simulink model "CrawlerValidation_Backup"  (R2018b)
settings: Solver=VariableStepAuto  StartTime=0.0  StopTime=10.0  RelTol=1e-3
model workspace: external: MAT-File C:\CrawlerValidation_DataFile1.mat (data not in the file)
undefined symbols (not defined in the file): smiData, X, Y, Z
libraries: sm_lib x20, nesl_utility x7
settings Model: Creator=Kim Jensen  LastModifiedBy=Kim Jensen

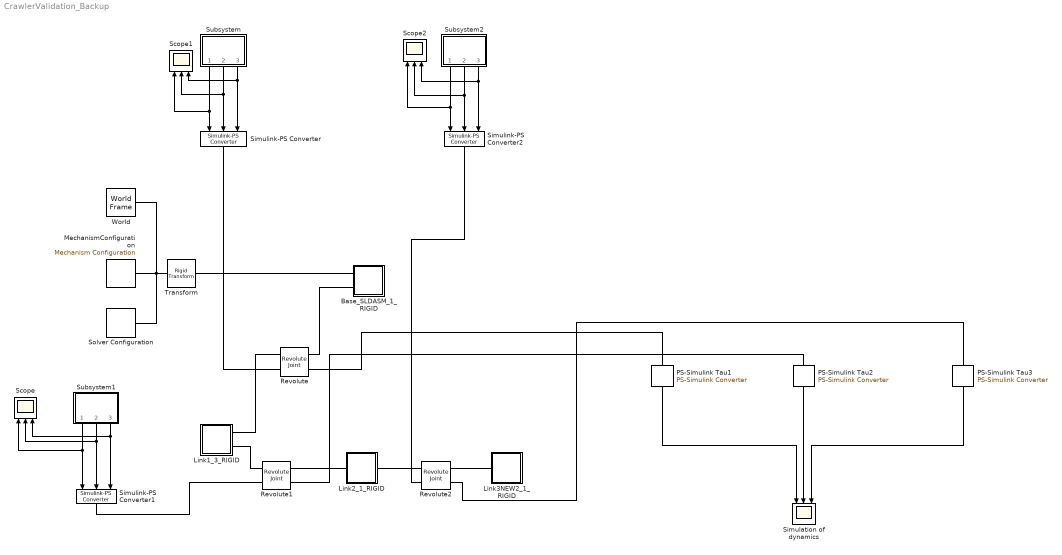
== system CrawlerValidation_Backup ==
  Base_SLDASM_1_RIGID : Subsystem
  Link1_3_RIGID : Subsystem
  Link2_1_RIGID : Subsystem
  Link3NEW2_1_RIGID : Subsystem
  MechanismConfiguration : sm_lib/Utilities/Mechanism Configuration  UniformGravity=Constant  GravityVector=[0 -9.80665 0]  GravityUnits=m/s^2  LinearizationDelta=0.001
  PS-Simulink Tau1 : nesl_utility/PS-Simulink Converter  PhysicalDomain=network_engine_domain  SubClassName=ps_output  LeftPortType=input  RightPortType=output  PseudoPeriodic=off  Frequencies=[]  Unit=1  AffineConversion=off
  PS-Simulink Tau2 : nesl_utility/PS-Simulink Converter  PhysicalDomain=network_engine_domain  SubClassName=ps_output  LeftPortType=input  RightPortType=output  PseudoPeriodic=off  Frequencies=[]  Unit=1  AffineConversion=off
  PS-Simulink Tau3 : nesl_utility/PS-Simulink Converter  PhysicalDomain=network_engine_domain  SubClassName=ps_output  LeftPortType=input  RightPortType=output  PseudoPeriodic=off  Frequencies=[]  Unit=1  AffineConversion=off
  Revolute : sm_lib/Joints/Revolute Joint  SenseConstraintForce=off  SenseConstraintForceX=off  SenseConstraintForceY=off  SenseConstraintForceZ=off  SenseConstraintTorque=off  SenseConstraintTorqueX=off  SenseConstraintTorqueY=off  SenseConstraintTorqueZ=off  SenseTotalForce=off  SenseTotalForceX=off  SenseTotalForceY=off  SenseTotalForceZ=off  SenseTotalTorque=off  SenseTotalTorqueX=off  SenseTotalTorqueY=off  SenseTotalTorqueZ=off  CompositeWrenchDir=FollowerOnBase  CompositeWrenchFrame=BaseFrame  EquilibriumPosition=0  EquilibriumPositionUnits=rad  SpringStiffness=0  SpringStiffnessUnits=N*m/rad  DampingCoefficient=0  DampingCoefficientUnits=N*m/(rad/s)  TorqueActuationMode=ComputedTorque  MotionActuationMode=InputMotion  SensePosition=off  SenseVelocity=off  SenseAcceleration=off  SenseTorqueForce=on  PositionTargetSpecify=on  PositionTargetPriority=Low  PositionTargetValue=smiData.RevoluteJoint(1).Rz.Pos  PositionTargetValueUnits=deg  VelocityTargetSpecify=off  VelocityTargetPriority=High  VelocityTargetValue=0  VelocityTargetValueUnits=deg/s
  Revolute1 : sm_lib/Joints/Revolute Joint  SenseConstraintForce=off  SenseConstraintForceX=off  SenseConstraintForceY=off  SenseConstraintForceZ=off  SenseConstraintTorque=off  SenseConstraintTorqueX=off  SenseConstraintTorqueY=off  SenseConstraintTorqueZ=off  SenseTotalForce=off  SenseTotalForceX=off  SenseTotalForceY=off  SenseTotalForceZ=off  SenseTotalTorque=off  SenseTotalTorqueX=off  SenseTotalTorqueY=off  SenseTotalTorqueZ=off  CompositeWrenchDir=FollowerOnBase  CompositeWrenchFrame=BaseFrame  EquilibriumPosition=0  EquilibriumPositionUnits=rad  SpringStiffness=0  SpringStiffnessUnits=N*m/rad  DampingCoefficient=0  DampingCoefficientUnits=N*m/(rad/s)  TorqueActuationMode=ComputedTorque  MotionActuationMode=InputMotion  SensePosition=off  SenseVelocity=off  SenseAcceleration=off  SenseTorqueForce=on  PositionTargetSpecify=on  PositionTargetPriority=Low  PositionTargetValue=smiData.RevoluteJoint(2).Rz.Pos  PositionTargetValueUnits=deg  VelocityTargetSpecify=off  VelocityTargetPriority=High  VelocityTargetValue=0  VelocityTargetValueUnits=deg/s
  Revolute2 : sm_lib/Joints/Revolute Joint  SenseConstraintForce=off  SenseConstraintForceX=off  SenseConstraintForceY=off  SenseConstraintForceZ=off  SenseConstraintTorque=off  SenseConstraintTorqueX=off  SenseConstraintTorqueY=off  SenseConstraintTorqueZ=off  SenseTotalForce=off  SenseTotalForceX=off  SenseTotalForceY=off  SenseTotalForceZ=off  SenseTotalTorque=off  SenseTotalTorqueX=off  SenseTotalTorqueY=off  SenseTotalTorqueZ=off  CompositeWrenchDir=FollowerOnBase  CompositeWrenchFrame=BaseFrame  EquilibriumPosition=0  EquilibriumPositionUnits=rad  SpringStiffness=0  SpringStiffnessUnits=N*m/rad  DampingCoefficient=0  DampingCoefficientUnits=N*m/(rad/s)  TorqueActuationMode=ComputedTorque  MotionActuationMode=InputMotion  SensePosition=off  SenseVelocity=off  SenseAcceleration=off  SenseTorqueForce=on  PositionTargetSpecify=on  PositionTargetPriority=Low  PositionTargetValue=smiData.RevoluteJoint(3).Rz.Pos  PositionTargetValueUnits=deg  VelocityTargetSpecify=off  VelocityTargetPriority=High  VelocityTargetValue=0  VelocityTargetValueUnits=deg/s
  Scope : Scope  NumInputPorts=3
  Scope1 : Scope  NumInputPorts=3
  Scope2 : Scope  NumInputPorts=3
  "Simulation of dynamics " : Scope  NumInputPorts=3
  Simulink-PS Converter : nesl_utility/Simulink-PS Converter  PhysicalDomain=network_engine_domain  SubClassName=ps_input  LeftPortType=input  RightPortType=output  PseudoPeriodic=off  Frequencies=[]  NoiseDistribution=none  NoiseParameters=[]  Unit=1  AffineConversion=off  FilteringAndDerivatives=provide  SimscapeFilterOrder=1  InputFilterTimeConstant=0.001  UdotUserProvided=2
  Simulink-PS Converter1 : nesl_utility/Simulink-PS Converter  PhysicalDomain=network_engine_domain  SubClassName=ps_input  LeftPortType=input  RightPortType=output  PseudoPeriodic=off  Frequencies=[]  NoiseDistribution=none  NoiseParameters=[]  Unit=1  AffineConversion=off  FilteringAndDerivatives=provide  SimscapeFilterOrder=1  InputFilterTimeConstant=0.001  UdotUserProvided=2
  Simulink-PS Converter2 : nesl_utility/Simulink-PS Converter  PhysicalDomain=network_engine_domain  SubClassName=ps_input  LeftPortType=input  RightPortType=output  PseudoPeriodic=off  Frequencies=[]  NoiseDistribution=none  NoiseParameters=[]  Unit=1  AffineConversion=off  FilteringAndDerivatives=provide  SimscapeFilterOrder=1  InputFilterTimeConstant=0.001  UdotUserProvided=2
  Solver Configuration : nesl_utility/Solver Configuration  PhysicalDomain=network_engine_domain  SubClassName=solver  LeftPortType=input  RightPortType=generic  Tones=[]  Harmonics=[]  SimulateNoise=off  Profile=off  UseLocalSampling=off  EnableSwitchedLinearOptims=on  FrequencyDomain=off  UseCCode=off  RelTol=0.001  AbsTol=1e-06  MinStep=1e-09  ToWorkspace=off  RevertToSquareIcSolve=off  NumHomotopyIterations=100  PhasorMode=off  PhasorModeNumHarmonics=1  DoDC=off  ResidualTolerance=1e-09  UseLocalSolver=off  LocalSolverChoice=NE_BACKWARD_EULER_ADVANCER  LocalSolverSampleTime=0.001  DoFixedCost=off  MaxNonlinIter=3  MaxModeIter=2  LinearAlgebra=auto  EquationFormulation=NE_TIME_EF  DelaysMemoryBudget=1024  AutomaticFiltering=on  FilteringTimeConstant=0.001  PartitionStorageMethod=AS_NEEDED  PartitionMemoryBudget=1024
  Subsystem : Subsystem
  Subsystem1 : Subsystem
  Subsystem2 : Subsystem
  Transform : sm_lib/Frames and Transforms/Rigid Transform  TranslationMethod=Cartesian  TranslationStandardOffset=0  TranslationLengthUnit=mm  TranslationStandardAxis=+Z  TranslationCartesianOffset=smiData.RigidTransform(7).translation  TranslationROffset=0  TranslationROffsetUnits=m  TranslationZOffset=0  TranslationZOffsetUnits=m  TranslationThetaOffset=0  TranslationThetaOffsetUnits=deg  RotationMethod=ArbitraryAxis  RotationAngleUnits=rad  RotationStandardAxis=+Z  RotationAngle=smiData.RigidTransform(7).angle  RotationArbitraryAxis=smiData.RigidTransform(7).axis  FollAlignAxisA=+X  BaseAlignAxisA=+Y  FollAlignAxisB=+Y  BaseAlignAxisB=+Z  RotationSequenceAxes=FollowerAxes  RotationSequence=XYX  RotationSequenceAngles=[0 0 0]  RotationSequenceAnglesUnits=deg  RotationMatrix=[1 0 0; 0 1 0; 0 0 1]
  World : sm_lib/Frames and Transforms/World Frame
  wires:
  Subsystem/3(ddtheta_1) -> Simulink-PS Converter/3, Scope1/3
  Subsystem2/2(dtheta_3) -> Simulink-PS Converter2/2, Scope2/2
  Subsystem2/3(ddtheta_3) -> Simulink-PS Converter2/3, Scope2/3
  Subsystem2/1(theta_3) -> Simulink-PS Converter2/1, Scope2/1
  Subsystem1/2(dtheta_2) -> Simulink-PS Converter1/2, Scope/2
  Subsystem1/3(ddtheta_2) -> Simulink-PS Converter1/3, Scope/3
  Subsystem1/1(theta_2) -> Simulink-PS Converter1/1, Scope/1
  PS-Simulink Tau1/1 -> "Simulation of dynamics "/1
  PS-Simulink Tau2/1 -> "Simulation of dynamics "/2
  PS-Simulink Tau3/1 -> "Simulation of dynamics "/3
  Subsystem/1(theta_1) -> Simulink-PS Converter/1, Scope1/1
  Subsystem/2(dtheta_1) -> Simulink-PS Converter/2, Scope1/2
  connections:
  Transform/LConn1 -- MechanismConfiguration/RConn1 -- Solver Configuration/RConn1 -- World/RConn1
  Base_SLDASM_1_RIGID/LConn1 -- Transform/RConn1
  Base_SLDASM_1_RIGID/LConn2 -- Revolute/RConn1
  Link1_3_RIGID/RConn1 -- Revolute/LConn1
  Simulink-PS Converter/RConn1 -- Revolute/LConn2
  PS-Simulink Tau1/LConn1 -- Revolute/RConn2
  Link2_1_RIGID/RConn1 -- Revolute2/LConn1
  Link3NEW2_1_RIGID/LConn1 -- Revolute2/RConn1
  PS-Simulink Tau3/LConn1 -- Revolute2/RConn2
  PS-Simulink Tau2/LConn1 -- Revolute1/RConn2
  Simulink-PS Converter1/RConn1 -- Revolute1/LConn2
  Link2_1_RIGID/LConn1 -- Revolute1/RConn1
  Link1_3_RIGID/RConn2 -- Revolute1/LConn1
  Simulink-PS Converter2/RConn1 -- Revolute2/LConn2

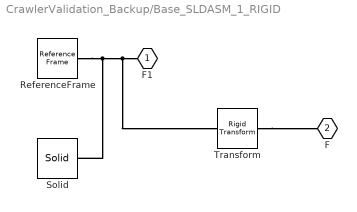
== system CrawlerValidation_Backup/Base_SLDASM_1_RIGID ==
  ReferenceFrame : sm_lib/Frames and Transforms/Reference Frame
  Solid : sm_lib/Body Elements/Solid  InertiaType=Custom  Mass=smiData.Solid(2).mass  MassUnits=kg  CenterOfMass=smiData.Solid(2).CoM  CenterOfMassUnits=mm  MomentsOfInertia=smiData.Solid(2).MoI  MomentsOfInertiaUnits=kg*mm^2  ProductsOfInertia=smiData.Solid(2).PoI  ProductsOfInertiaUnits=kg*mm^2  BasedOnType=Density  Density=1000  DensityUnits=kg/m^3  DoExposeReferenceFrame=on  SerializedFrames=<Frames/>  GraphicType=FromGeometry  MarkerShape=Sphere  MarkerSize=10  GraphicVisPropType=SimpleVisualProperties  GraphicDiffuseColor=smiData.Solid(2).color  GraphicSpecularColor=[0.5 0.5 0.5 1.0]  GraphicAmbientColor=[0.15 0.15 0.15 1.0]  GraphicEmissiveColor=[0.0 0.0 0.0 1.0]  GraphicShininess=75  GraphicOpacity=smiData.Solid(2).opacity  GeometryShape=FromFile  RectangleSize=[1 1]  RectangleSizeUnits=m  BrickDimensions=[1 1 1]  BrickDimensionUnits=m  CylinderRadius=1  CylinderRadiusUnits=m  CylinderLength=1  CylinderLengthUnits=m  SphereRadius=1  SphereRadiusUnits=m  EllipsoidRadii=[1 1 1]  EllipsoidRadiiUnits=m  ExtrusionCrossSection=[1 1; -1 1; -1 -1; 1 -1]  ExtrusionCrossSectionUnits=m  ExtrusionLength=1  ExtrusionLengthUnits=m  PolygonNumSides=3  PolygonOuterRadius=1  PolygonOuterRadiusUnits=m  ExtGeomFileType=STEP  ExtGeomFileName=Base.SLDASM_Default_sldprt.STEP  ExtGeomFileUnits=m  RevolutionCrossSection=[1 1; 1 -1; 2 -1; 2 1]  RevolutionCrossSectionUnits=m  RevolutionExtent=Full  RevolutionAngle=180  RevolutionAngleUnits=deg
  Transform : sm_lib/Frames and Transforms/Rigid Transform  TranslationMethod=Cartesian  TranslationStandardOffset=0  TranslationLengthUnit=mm  TranslationStandardAxis=+Z  TranslationCartesianOffset=smiData.RigidTransform(6).translation  TranslationROffset=0  TranslationROffsetUnits=m  TranslationZOffset=0  TranslationZOffsetUnits=m  TranslationThetaOffset=0  TranslationThetaOffsetUnits=deg  RotationMethod=ArbitraryAxis  RotationAngleUnits=rad  RotationStandardAxis=+Z  RotationAngle=smiData.RigidTransform(6).angle  RotationArbitraryAxis=smiData.RigidTransform(6).axis  FollAlignAxisA=+X  BaseAlignAxisA=+Y  FollAlignAxisB=+Y  BaseAlignAxisB=+Z  RotationSequenceAxes=FollowerAxes  RotationSequence=XYX  RotationSequenceAngles=[0 0 0]  RotationSequenceAnglesUnits=deg  RotationMatrix=[1 0 0; 0 1 0; 0 0 1]
  F1 : PMIOPort  Side=Left
  F : PMIOPort  Port=2  Side=Left
  connections:
  Solid/RConn1 -- ReferenceFrame/RConn1 -- Transform/LConn1 -- F1/RConn1
  Transform/RConn1 -- F/RConn1

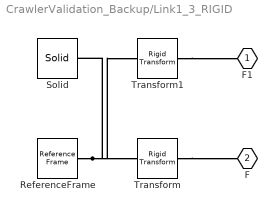
== system CrawlerValidation_Backup/Link1_3_RIGID ==
  ReferenceFrame : sm_lib/Frames and Transforms/Reference Frame
  Solid : sm_lib/Body Elements/Solid  InertiaType=Custom  Mass=smiData.Solid(1).mass  MassUnits=kg  CenterOfMass=smiData.Solid(1).CoM  CenterOfMassUnits=mm  MomentsOfInertia=smiData.Solid(1).MoI  MomentsOfInertiaUnits=kg*mm^2  ProductsOfInertia=smiData.Solid(1).PoI  ProductsOfInertiaUnits=kg*mm^2  BasedOnType=Density  Density=1000  DensityUnits=kg/m^3  DoExposeReferenceFrame=on  SerializedFrames=<Frames/>  GraphicType=FromGeometry  MarkerShape=Sphere  MarkerSize=10  GraphicVisPropType=SimpleVisualProperties  GraphicDiffuseColor=smiData.Solid(1).color  GraphicSpecularColor=[0.5 0.5 0.5 1.0]  GraphicAmbientColor=[0.15 0.15 0.15 1.0]  GraphicEmissiveColor=[0.0 0.0 0.0 1.0]  GraphicShininess=75  GraphicOpacity=smiData.Solid(1).opacity  GeometryShape=FromFile  RectangleSize=[1 1]  RectangleSizeUnits=m  BrickDimensions=[1 1 1]  BrickDimensionUnits=m  CylinderRadius=1  CylinderRadiusUnits=m  CylinderLength=1  CylinderLengthUnits=m  SphereRadius=1  SphereRadiusUnits=m  EllipsoidRadii=[1 1 1]  EllipsoidRadiiUnits=m  ExtrusionCrossSection=[1 1; -1 1; -1 -1; 1 -1]  ExtrusionCrossSectionUnits=m  ExtrusionLength=1  ExtrusionLengthUnits=m  PolygonNumSides=3  PolygonOuterRadius=1  PolygonOuterRadiusUnits=m  ExtGeomFileType=STEP  ExtGeomFileName=Link1_Default_sldprt.STEP  ExtGeomFileUnits=m  RevolutionCrossSection=[1 1; 1 -1; 2 -1; 2 1]  RevolutionCrossSectionUnits=m  RevolutionExtent=Full  RevolutionAngle=180  RevolutionAngleUnits=deg
  Transform : sm_lib/Frames and Transforms/Rigid Transform  TranslationMethod=Cartesian  TranslationStandardOffset=0  TranslationLengthUnit=mm  TranslationStandardAxis=+Z  TranslationCartesianOffset=smiData.RigidTransform(1).translation  TranslationROffset=0  TranslationROffsetUnits=m  TranslationZOffset=0  TranslationZOffsetUnits=m  TranslationThetaOffset=0  TranslationThetaOffsetUnits=deg  RotationMethod=ArbitraryAxis  RotationAngleUnits=rad  RotationStandardAxis=+Z  RotationAngle=smiData.RigidTransform(1).angle  RotationArbitraryAxis=smiData.RigidTransform(1).axis  FollAlignAxisA=+X  BaseAlignAxisA=+Y  FollAlignAxisB=+Y  BaseAlignAxisB=+Z  RotationSequenceAxes=FollowerAxes  RotationSequence=XYX  RotationSequenceAngles=[0 0 0]  RotationSequenceAnglesUnits=deg  RotationMatrix=[1 0 0; 0 1 0; 0 0 1]
  Transform1 : sm_lib/Frames and Transforms/Rigid Transform  TranslationMethod=Cartesian  TranslationStandardOffset=0  TranslationLengthUnit=mm  TranslationStandardAxis=+Z  TranslationCartesianOffset=smiData.RigidTransform(5).translation  TranslationROffset=0  TranslationROffsetUnits=m  TranslationZOffset=0  TranslationZOffsetUnits=m  TranslationThetaOffset=0  TranslationThetaOffsetUnits=deg  RotationMethod=ArbitraryAxis  RotationAngleUnits=rad  RotationStandardAxis=+Z  RotationAngle=smiData.RigidTransform(5).angle  RotationArbitraryAxis=smiData.RigidTransform(5).axis  FollAlignAxisA=+X  BaseAlignAxisA=+Y  FollAlignAxisB=+Y  BaseAlignAxisB=+Z  RotationSequenceAxes=FollowerAxes  RotationSequence=XYX  RotationSequenceAngles=[0 0 0]  RotationSequenceAnglesUnits=deg  RotationMatrix=[1 0 0; 0 1 0; 0 0 1]
  F1 : PMIOPort  Side=Right
  F : PMIOPort  Port=2  Side=Right
  connections:
  Solid/RConn1 -- ReferenceFrame/RConn1 -- Transform/LConn1 -- Transform1/LConn1
  Transform/RConn1 -- F/RConn1
  Transform1/RConn1 -- F1/RConn1

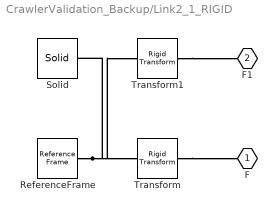
== system CrawlerValidation_Backup/Link2_1_RIGID ==
  ReferenceFrame : sm_lib/Frames and Transforms/Reference Frame
  Solid : sm_lib/Body Elements/Solid  InertiaType=Custom  Mass=smiData.Solid(3).mass  MassUnits=kg  CenterOfMass=smiData.Solid(3).CoM  CenterOfMassUnits=mm  MomentsOfInertia=smiData.Solid(3).MoI  MomentsOfInertiaUnits=kg*mm^2  ProductsOfInertia=smiData.Solid(3).PoI  ProductsOfInertiaUnits=kg*mm^2  BasedOnType=Density  Density=1000  DensityUnits=kg/m^3  DoExposeReferenceFrame=on  SerializedFrames=<Frames/>  GraphicType=FromGeometry  MarkerShape=Sphere  MarkerSize=10  GraphicVisPropType=SimpleVisualProperties  GraphicDiffuseColor=smiData.Solid(3).color  GraphicSpecularColor=[0.5 0.5 0.5 1.0]  GraphicAmbientColor=[0.15 0.15 0.15 1.0]  GraphicEmissiveColor=[0.0 0.0 0.0 1.0]  GraphicShininess=75  GraphicOpacity=smiData.Solid(3).opacity  GeometryShape=FromFile  RectangleSize=[1 1]  RectangleSizeUnits=m  BrickDimensions=[1 1 1]  BrickDimensionUnits=m  CylinderRadius=1  CylinderRadiusUnits=m  CylinderLength=1  CylinderLengthUnits=m  SphereRadius=1  SphereRadiusUnits=m  EllipsoidRadii=[1 1 1]  EllipsoidRadiiUnits=m  ExtrusionCrossSection=[1 1; -1 1; -1 -1; 1 -1]  ExtrusionCrossSectionUnits=m  ExtrusionLength=1  ExtrusionLengthUnits=m  PolygonNumSides=3  PolygonOuterRadius=1  PolygonOuterRadiusUnits=m  ExtGeomFileType=STEP  ExtGeomFileName=Link2_Default_sldprt.STEP  ExtGeomFileUnits=m  RevolutionCrossSection=[1 1; 1 -1; 2 -1; 2 1]  RevolutionCrossSectionUnits=m  RevolutionExtent=Full  RevolutionAngle=180  RevolutionAngleUnits=deg
  Transform : sm_lib/Frames and Transforms/Rigid Transform  TranslationMethod=Cartesian  TranslationStandardOffset=0  TranslationLengthUnit=mm  TranslationStandardAxis=+Z  TranslationCartesianOffset=smiData.RigidTransform(2).translation  TranslationROffset=0  TranslationROffsetUnits=m  TranslationZOffset=0  TranslationZOffsetUnits=m  TranslationThetaOffset=0  TranslationThetaOffsetUnits=deg  RotationMethod=ArbitraryAxis  RotationAngleUnits=rad  RotationStandardAxis=+Z  RotationAngle=smiData.RigidTransform(2).angle  RotationArbitraryAxis=smiData.RigidTransform(2).axis  FollAlignAxisA=+X  BaseAlignAxisA=+Y  FollAlignAxisB=+Y  BaseAlignAxisB=+Z  RotationSequenceAxes=FollowerAxes  RotationSequence=XYX  RotationSequenceAngles=[0 0 0]  RotationSequenceAnglesUnits=deg  RotationMatrix=[1 0 0; 0 1 0; 0 0 1]
  Transform1 : sm_lib/Frames and Transforms/Rigid Transform  TranslationMethod=Cartesian  TranslationStandardOffset=0  TranslationLengthUnit=mm  TranslationStandardAxis=+Z  TranslationCartesianOffset=smiData.RigidTransform(3).translation  TranslationROffset=0  TranslationROffsetUnits=m  TranslationZOffset=0  TranslationZOffsetUnits=m  TranslationThetaOffset=0  TranslationThetaOffsetUnits=deg  RotationMethod=ArbitraryAxis  RotationAngleUnits=rad  RotationStandardAxis=+Z  RotationAngle=smiData.RigidTransform(3).angle  RotationArbitraryAxis=smiData.RigidTransform(3).axis  FollAlignAxisA=+X  BaseAlignAxisA=+Y  FollAlignAxisB=+Y  BaseAlignAxisB=+Z  RotationSequenceAxes=FollowerAxes  RotationSequence=XYX  RotationSequenceAngles=[0 0 0]  RotationSequenceAnglesUnits=deg  RotationMatrix=[1 0 0; 0 1 0; 0 0 1]
  F : PMIOPort  Side=Left
  F1 : PMIOPort  Port=2  Side=Right
  connections:
  Solid/RConn1 -- ReferenceFrame/RConn1 -- Transform/LConn1 -- Transform1/LConn1
  Transform/RConn1 -- F/RConn1
  Transform1/RConn1 -- F1/RConn1

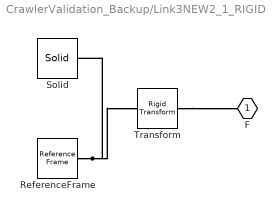
== system CrawlerValidation_Backup/Link3NEW2_1_RIGID ==
  ReferenceFrame : sm_lib/Frames and Transforms/Reference Frame
  Solid : sm_lib/Body Elements/Solid  InertiaType=Custom  Mass=smiData.Solid(4).mass  MassUnits=kg  CenterOfMass=smiData.Solid(4).CoM  CenterOfMassUnits=mm  MomentsOfInertia=smiData.Solid(4).MoI  MomentsOfInertiaUnits=kg*mm^2  ProductsOfInertia=smiData.Solid(4).PoI  ProductsOfInertiaUnits=kg*mm^2  BasedOnType=Density  Density=1000  DensityUnits=kg/m^3  DoExposeReferenceFrame=on  SerializedFrames=<Frames/>  GraphicType=FromGeometry  MarkerShape=Sphere  MarkerSize=10  GraphicVisPropType=SimpleVisualProperties  GraphicDiffuseColor=smiData.Solid(4).color  GraphicSpecularColor=[0.5 0.5 0.5 1.0]  GraphicAmbientColor=[0.15 0.15 0.15 1.0]  GraphicEmissiveColor=[0.0 0.0 0.0 1.0]  GraphicShininess=75  GraphicOpacity=smiData.Solid(4).opacity  GeometryShape=FromFile  RectangleSize=[1 1]  RectangleSizeUnits=m  BrickDimensions=[1 1 1]  BrickDimensionUnits=m  CylinderRadius=1  CylinderRadiusUnits=m  CylinderLength=1  CylinderLengthUnits=m  SphereRadius=1  SphereRadiusUnits=m  EllipsoidRadii=[1 1 1]  EllipsoidRadiiUnits=m  ExtrusionCrossSection=[1 1; -1 1; -1 -1; 1 -1]  ExtrusionCrossSectionUnits=m  ExtrusionLength=1  ExtrusionLengthUnits=m  PolygonNumSides=3  PolygonOuterRadius=1  PolygonOuterRadiusUnits=m  ExtGeomFileType=STEP  ExtGeomFileName=Link3NEW2_Default_sldprt.STEP  ExtGeomFileUnits=m  RevolutionCrossSection=[1 1; 1 -1; 2 -1; 2 1]  RevolutionCrossSectionUnits=m  RevolutionExtent=Full  RevolutionAngle=180  RevolutionAngleUnits=deg
  Transform : sm_lib/Frames and Transforms/Rigid Transform  TranslationMethod=Cartesian  TranslationStandardOffset=0  TranslationLengthUnit=mm  TranslationStandardAxis=+Z  TranslationCartesianOffset=smiData.RigidTransform(4).translation  TranslationROffset=0  TranslationROffsetUnits=m  TranslationZOffset=0  TranslationZOffsetUnits=m  TranslationThetaOffset=0  TranslationThetaOffsetUnits=deg  RotationMethod=ArbitraryAxis  RotationAngleUnits=rad  RotationStandardAxis=+Z  RotationAngle=smiData.RigidTransform(4).angle  RotationArbitraryAxis=smiData.RigidTransform(4).axis  FollAlignAxisA=+X  BaseAlignAxisA=+Y  FollAlignAxisB=+Y  BaseAlignAxisB=+Z  RotationSequenceAxes=FollowerAxes  RotationSequence=XYX  RotationSequenceAngles=[0 0 0]  RotationSequenceAnglesUnits=deg  RotationMatrix=[1 0 0; 0 1 0; 0 0 1]
  F : PMIOPort  Side=Left
  connections:
  Solid/RConn1 -- ReferenceFrame/RConn1 -- Transform/LConn1
  Transform/RConn1 -- F/RConn1

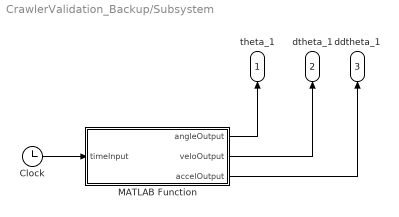
== system CrawlerValidation_Backup/Subsystem ==
  Clock : Clock
  MATLAB Function : MATLAB Function  TreatAsAtomicUnit=on
  theta_1 : Outport
  dtheta_1 : Outport  Port=2
  ddtheta_1 : Outport  Port=3
  wires:
  MATLAB Function/3(accelOutput) -> ddtheta_1/1
  MATLAB Function/2(veloOutput) -> dtheta_1/1
  MATLAB Function/1(angleOutput) -> theta_1/1
  Clock/1 -> MATLAB Function/1(timeInput)

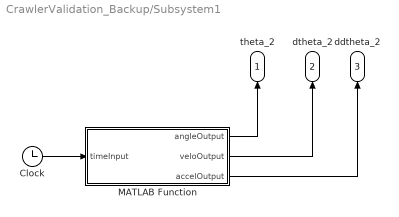
== system CrawlerValidation_Backup/Subsystem1 ==
  Clock : Clock
      settings: Decimation=1000
  MATLAB Function : MATLAB Function  TreatAsAtomicUnit=on
  theta_2 : Outport
  dtheta_2 : Outport  Port=2
  ddtheta_2 : Outport  Port=3
  wires:
  MATLAB Function/3(accelOutput) -> ddtheta_2/1
  MATLAB Function/2(veloOutput) -> dtheta_2/1
  MATLAB Function/1(angleOutput) -> theta_2/1
  Clock/1 -> MATLAB Function/1(timeInput)

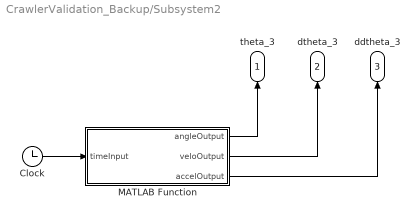
== system CrawlerValidation_Backup/Subsystem2 ==
  Clock : Clock
  MATLAB Function : MATLAB Function  TreatAsAtomicUnit=on
  theta_3 : Outport
  dtheta_3 : Outport  Port=2
  ddtheta_3 : Outport  Port=3
  wires:
  MATLAB Function/3(accelOutput) -> ddtheta_3/1
  MATLAB Function/2(veloOutput) -> dtheta_3/1
  MATLAB Function/1(angleOutput) -> theta_3/1
  Clock/1 -> MATLAB Function/1(timeInput)

== matlab function CrawlerValidation_Backup/Subsystem1/MATLAB Function ==
  data: timeInput input; angleOutput output; veloOutput output; accelOutput output
function [angleOutput,veloOutput,accelOutput] = TrajectoryJoint2(timeInput)  
theta0 = -40*pi/180;
thetaf = -40*pi/180;
%Lengths of bodies
L2 = 0.2185;
L3 = 0.1456;
%Masses of bodies
M2 = 0.228;
M3 = 0.303;
%mass of object held
M = 0;
%Time between start and stop (dependent on gesture)
t = 2;
%Mass in kg
m = M+M2+M3; 

%Stopping distance
d = 0.002;

%Max allowed force
F = 35;

%Force of impact
% F = (0.5 * m * v^2) ? d

%Max speed in m/s
v = (sqrt(2)*sqrt(d)*sqrt(F))/sqrt(m);

%Length of the arm moving in m

r = L2+L3;

%Angular max speed in rad/s

omega = v/r

%Acceleration time in seconds
ta = 0.05;


%Acceleration for the given speed if accelerating for ta seconds
a = omega/ta

%%%%%%%%%%%%%%%%%
%PARABOLIC BLEND%
%%%%%%%%%%%%%%%%%

%Time of movement
time = 0:.005:t; 


%Calculating tb (Time when speed is constant
tb = (t/2) - (sqrt((a.^2)*(t.^2)-4*a*(thetaf-theta0)))/(2*a);

%Angle when speed is constant
thetab = (1/2)*a*tb.^2+theta0;

%Acceleration to need speed
acc = theta0+(1/2)*a*time.^2;

%Constant Speed
const = thetab+a*tb*(time-tb);

%Deacceleration
deacc = thetaf - ((1/2)*a*(t-time).^2);

%Velocity functions
vAcc = diff(acc)./diff(time);
vConst = diff(const)./diff(time);
vDeacc = diff(deacc)./diff(time);

%Intervals for plotting
accInt = (time>=0 & time <=tb);
constInt = (time>=tb & time <=t-tb);
deaccInt = (time>=t-tb & time<t);

% if(timeInput>=0 & timeInput<=tb)
%     angleOutput = theta0 + 1/2*a*timeInput^2;
%     veloOutput = omega-a*(tb-timeInput);
%     accelOutput = a;
% elseif (timeInput>=tb & timeInput<=t-tb)
%     angleOutput = theta0 + a*tb*(timeInput-tb);
%     veloOutput = omega;
%     accelOutput = 0;
% elseif (timeInput>=t-tb & timeInput<t)
%     angleOutput = thetaf-1/2*a*(t-timeInput)^2;
%     veloOutput = omega-a*(t-tb-timeInput);
%     accelOutput = -a ;
% else
%     angleOutput = thetaf;
%     veloOutput = 0;
%     accelOutput = 0;
%     
% end

angleOutput = thetaf;
 veloOutput = 0;
accelOutput = 0;

== matlab function CrawlerValidation_Backup/Subsystem/MATLAB Function ==
  data: timeInput input; angleOutput output; veloOutput output; accelOutput output
function [angleOutput,veloOutput,accelOutput] = TrajectoryJoint1(timeInput)  
theta0 = -40*pi/180;
thetaf = 0;
%Lengths of bodies
L2 = 0.2185;
L3 = 0.1456;
%Masses of bodies
M2 = 0.228;
M3 = 0.303;
%mass of object held
M = 0;
%Time between start and stop (dependent on gesture)
t = 2;
%Mass in kg
m = M+M2+M3; 

%Stopping distance
d = 0.002;

%Max allowed force
F = 35;

%Force of impact
% F = (0.5 * m * v^2) ? d

%Max speed in m/s
v = (sqrt(2)*sqrt(d)*sqrt(F))/sqrt(m);

%Length of the arm moving in m

r = L2+L3;

%Angular max speed in rad/s

omega = v/r

%Acceleration time in seconds
ta = 0.05;


%Acceleration for the given speed if accelerating for ta seconds
a = omega/ta

%%%%%%%%%%%%%%%%%
%PARABOLIC BLEND%
%%%%%%%%%%%%%%%%%

%Time of movement
time = 0:.005:t; 


%Calculating tb (Time when speed is constant
tb = (t/2) - (sqrt((a.^2)*(t.^2)-4*a*(thetaf-theta0)))/(2*a);

%Angle when speed is constant
thetab = (1/2)*a*tb.^2+theta0;

%Acceleration to need speed
acc = theta0+(1/2)*a*time.^2;

%Constant Speed
const = thetab+a*tb*(time-tb);

%Deacceleration
deacc = thetaf - ((1/2)*a*(t-time).^2);

%Velocity functions
vAcc = diff(acc)./diff(time);
vConst = diff(const)./diff(time);
vDeacc = diff(deacc)./diff(time);

%Intervals for plotting
accInt = (time>=0 & time <=tb);
constInt = (time>=tb & time <=t-tb);
deaccInt = (time>=t-tb & time<t);

% if(timeInput>=0 & timeInput<=tb)
%     angleOutput = theta0 + 1/2*a*timeInput^2;
%     veloOutput = omega-a*(tb-timeInput);
%     accelOutput = a;
% elseif (timeInput>=tb & timeInput<=t-tb)
%     angleOutput = theta0 + a*tb*(timeInput-tb);
%     veloOutput = omega;
%     accelOutput = 0;
% elseif (timeInput>=t-tb & timeInput<t)
%     angleOutput = thetaf-1/2*a*(t-timeInput)^2;
%     veloOutput = omega-a*(t-tb-timeInput);
%     accelOutput = -a ;
% else
%     angleOutput = thetaf;
%     veloOutput = 0;
%     accelOutput = 0;
%     
% end

angleOutput = thetaf;
 veloOutput = 0;
accelOutput = 0;

== matlab function CrawlerValidation_Backup/Subsystem2/MATLAB Function ==
  data: timeInput input; angleOutput output; veloOutput output; accelOutput output
function [angleOutput,veloOutput,accelOutput] = TrajectoryJoint3(timeInput)  
theta0 = 0;
thetaf = -2.8;
%Lengths of bodies

L3 = 0.1456;
%Masses of bodies

M3 = 0.303;
%mass of object held
M = 0;
%Time between start and stop (dependent on gesture)
t = 2;
%Mass in kg
m = M+M3; 

%Stopping distance
d = 0.002;

%Max allowed force
F = 35;

%Force of impact
% F = (0.5 * m * v^2) ? d

%Max speed in m/s
v = (sqrt(2)*sqrt(d)*sqrt(F))/sqrt(m);

%Length of the arm moving in m

r = L3;

%Angular max speed in rad/s

omega = v/r

%Acceleration time in seconds
ta = 0.05;


%Acceleration for the given speed if accelerating for ta seconds
a = omega/ta

%%%%%%%%%%%%%%%%%
%PARABOLIC BLEND%
%%%%%%%%%%%%%%%%%

%Time of movement
time = 0:.005:t; 


%Calculating tb (Time when speed is constant
tb = (t/2) - (sqrt((a.^2)*(t.^2)-4*a*(thetaf-theta0)))/(2*a);

%Angle when speed is constant
thetab = (1/2)*a*tb.^2+theta0;

%Acceleration to need speed
acc = theta0+(1/2)*a*time.^2;

%Constant Speed
const = thetab+a*tb*(time-tb);

%Deacceleration
deacc = thetaf - ((1/2)*a*(t-time).^2);

%Velocity functions
vAcc = diff(acc)./diff(time);
vConst = diff(const)./diff(time);
vDeacc = diff(deacc)./diff(time);

%Intervals for plotting
accInt = (time>=0 & time <=tb);
constInt = (time>=tb & time <=t-tb);
deaccInt = (time>=t-tb & time<t);

% if(timeInput>=0 & timeInput<=tb)
%     angleOutput = theta0 + 1/2*a*timeInput^2;
%     veloOutput = omega-a*(tb-timeInput);
%     accelOutput = a;
% elseif (timeInput>=tb & timeInput<=t-tb)
%     angleOutput = theta0 + a*tb*(timeInput-tb);
%     veloOutput = omega;
%     accelOutput = 0;
% elseif (timeInput>=t-tb & timeInput<t)
%     angleOutput = thetaf-1/2*a*(t-timeInput)^2;
%     veloOutput = omega-a*(t-tb-timeInput);
%     accelOutput = -a ;
% else
%     angleOutput = thetaf;
%     veloOutput = 0;
%     accelOutput = 0;
%     
% end

angleOutput = thetaf;
 veloOutput = 0;
accelOutput = 0;
